simulink model "svpwm"  (R2018a)
settings: Solver=VariableStepDiscrete  StartTime=0.0  StopTime=3  RelTol=1e-3
undefined symbols (not defined in the file): DiscIntNeverNeededParam
libraries: powerlib x16, simulink x3, powerlib_meascontrol x2
settings Model: Creator=HP  LastModifiedBy=HP
settings SolverCC: ZeroCrossAlgorithm=Adaptive
settings DebuggingCC: MaxConsecutiveZCsMsg=none

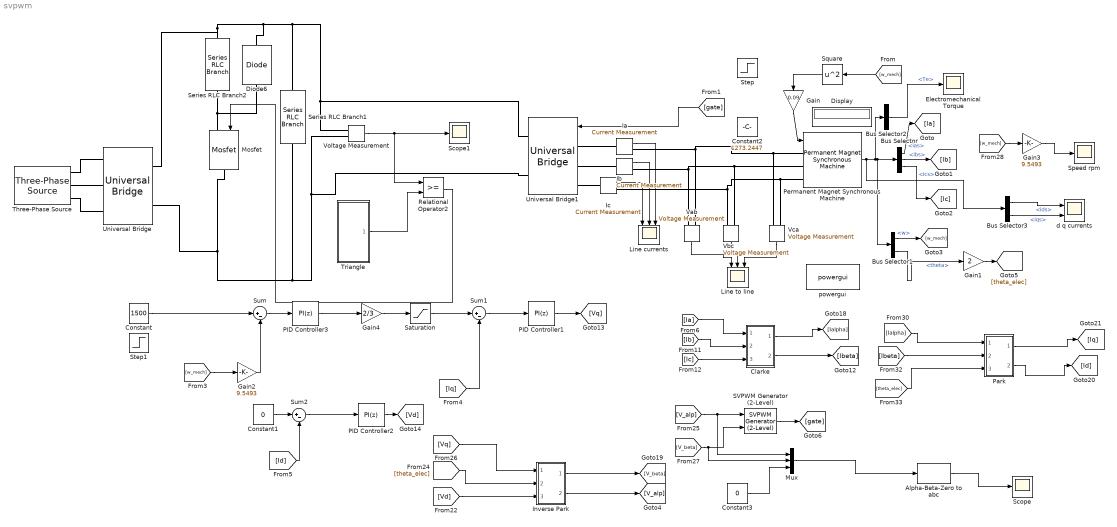
== system svpwm ==
  Alpha-Beta-Zero to abc : powerlib_meascontrol/Transformations/Alpha-Beta-Zero to abc
      settings: SourceProductName=Simscape Power Systems  SourceProductBaseCode=PS
  Bus Selector : BusSelector  OutputSignals=ias,ibs,ics
  Bus Selector1 : BusSelector  OutputSignals=w,theta
  Bus Selector2 : BusSelector  OutputSignals=Te
  Bus Selector3 : BusSelector  OutputSignals=ids,iqs
  Clarke : Subsystem
  Constant : Constant  Value=1500
  Constant1 : Constant  Value=0
  Constant2 : Constant  Value=1273.2447
  Constant3 : Constant  Value=0
  Diode6 : powerlib/Power Electronics/Diode  Ron=0.001  Lon=0  Vf=1  IC=0  UseSnubber=0  Rs=500  Cs=250e-9  Measurements=off
  Display : Display
  Electromechanical Torque : Scope
  Gain : Gain  Gain=0.09
  Gain1 : Gain  Gain=2
  Gain2 : Gain  Gain=9.5493
  Gain3 : Gain  Gain=9.5493
  Gain4 : Gain  Gain=2/3
  Ia : powerlib/Measurements/Current Measurement  PhasorSimulation=off  OutputType=Complex  PSBequivalent=0
  Ib : powerlib/Measurements/Current Measurement  PhasorSimulation=off  OutputType=Complex  PSBequivalent=0
  Ic : powerlib/Measurements/Current Measurement  PhasorSimulation=off  OutputType=Complex  PSBequivalent=0
  Inverse Park : Subsystem
  Line currents : Scope  NumInputPorts=3
  Line to line : Scope  NumInputPorts=3
  Mosfet : powerlib/Power Electronics/Mosfet  Ron=0.1  Lon=0  Rd=0.025  Vfd=0  IC=0  Rs=1e5  Cs=inf  Measurements=off
  Mux : Mux  Inputs=3
  PID Controller1 : simulink/Continuous/PID Controller  Controller=PI  TimeDomain=Discrete-time  SampleTime=-1  IntegratorMethod=Forward Euler  FilterMethod=Forward Euler  Form=Parallel  UseFilter=on  ControllerParametersSource=internal  P=0.1  I=1000  D=0  N=100  InitialConditionSource=internal  InitialConditionForIntegrator=0  InitialConditionForFilter=0  ExternalReset=none  LimitOutput=off  UpperSaturationLimit=inf  LowerSaturationLimit=-inf  LinearizeAsGain=on  AntiWindupMode=none  Kb=1  TrackingMode=off  Kt=1  PParamMin=[]  PParamMax=[]  IParamMin=[]  IParamMax=[]  DParamMin=[]  DParamMax=[]  NParamMin=[]  NParamMax=[]  KbParamMin=[]  KbParamMax=[]  KtParamMin=[]  KtParamMax=[]  POutMin=[]  POutMax=[]  IOutMin=[]  IOutMax=[]  DOutMin=[]  DOutMax=[]  NOutMin=[]  NOutMax=[]  KbOutMin=[]  KbOutMax=[]  KtOutMin=[]  KtOutMax=[]  IntegratorOutMin=[]  IntegratorOutMax=[]  FilterOutMin=[]  FilterOutMax=[]  SumOutMin=[]  SumOutMax=[]  SumI1OutMin=[]  SumI1OutMax=[]  SumI2OutMin=[]  SumI2OutMax=[]  SumI3OutMin=[]  SumI3OutMax=[]  SumDOutMin=[]  SumDOutMax=[]  SaturationOutMin=[]  SaturationOutMax=[]  IntegratorContinuousStateAttributes=''  IntegratorStateMustResolveToSignalObject=off  IntegratorRTWStateStorageClass=Auto  FilterContinuousStateAttributes=''  FilterStateMustResolveToSignalObject=off  FilterRTWStateStorageClass=Auto  DifferentiatorICPrevScaledInput=0  DifferentiatorOutMin=[]  DifferentiatorOutMax=[]  FilterDiffOutCoefMin=[]  FilterDiffOutCoefMax=[]  SumDenOutMin=[]  SumDenOutMax=[]  SumNumOutMin=[]  SumNumOutMax=[]  ReciprocalOutMin=[]  ReciprocalOutMax=[]  DivideOutMin=[]  DivideOutMax=[]  TunerSelectOption=Transfer Function Based (PID Tuner App)
  PID Controller2 : simulink/Continuous/PID Controller  Controller=PI  TimeDomain=Discrete-time  SampleTime=-1  IntegratorMethod=Forward Euler  FilterMethod=Forward Euler  Form=Parallel  UseFilter=on  ControllerParametersSource=internal  P=0.1  I=1000  D=0  N=100  InitialConditionSource=internal  InitialConditionForIntegrator=0  InitialConditionForFilter=0  ExternalReset=none  LimitOutput=off  UpperSaturationLimit=inf  LowerSaturationLimit=-inf  LinearizeAsGain=on  AntiWindupMode=none  Kb=1  TrackingMode=off  Kt=1  PParamMin=[]  PParamMax=[]  IParamMin=[]  IParamMax=[]  DParamMin=[]  DParamMax=[]  NParamMin=[]  NParamMax=[]  KbParamMin=[]  KbParamMax=[]  KtParamMin=[]  KtParamMax=[]  POutMin=[]  POutMax=[]  IOutMin=[]  IOutMax=[]  DOutMin=[]  DOutMax=[]  NOutMin=[]  NOutMax=[]  KbOutMin=[]  KbOutMax=[]  KtOutMin=[]  KtOutMax=[]  IntegratorOutMin=[]  IntegratorOutMax=[]  FilterOutMin=[]  FilterOutMax=[]  SumOutMin=[]  SumOutMax=[]  SumI1OutMin=[]  SumI1OutMax=[]  SumI2OutMin=[]  SumI2OutMax=[]  SumI3OutMin=[]  SumI3OutMax=[]  SumDOutMin=[]  SumDOutMax=[]  SaturationOutMin=[]  SaturationOutMax=[]  IntegratorContinuousStateAttributes=''  IntegratorStateMustResolveToSignalObject=off  IntegratorRTWStateStorageClass=Auto  FilterContinuousStateAttributes=''  FilterStateMustResolveToSignalObject=off  FilterRTWStateStorageClass=Auto  DifferentiatorICPrevScaledInput=0  DifferentiatorOutMin=[]  DifferentiatorOutMax=[]  FilterDiffOutCoefMin=[]  FilterDiffOutCoefMax=[]  SumDenOutMin=[]  SumDenOutMax=[]  SumNumOutMin=[]  SumNumOutMax=[]  ReciprocalOutMin=[]  ReciprocalOutMax=[]  DivideOutMin=[]  DivideOutMax=[]  TunerSelectOption=Transfer Function Based (PID Tuner App)
  PID Controller3 : simulink/Continuous/PID Controller  Controller=PI  TimeDomain=Discrete-time  SampleTime=-1  IntegratorMethod=Forward Euler  FilterMethod=Forward Euler  Form=Parallel  UseFilter=on  ControllerParametersSource=internal  P=1000  I=1  D=0  N=100  InitialConditionSource=internal  InitialConditionForIntegrator=0  InitialConditionForFilter=0  ExternalReset=none  LimitOutput=off  UpperSaturationLimit=inf  LowerSaturationLimit=-inf  LinearizeAsGain=on  AntiWindupMode=none  Kb=1  TrackingMode=off  Kt=1  PParamMin=[]  PParamMax=[]  IParamMin=[]  IParamMax=[]  DParamMin=[]  DParamMax=[]  NParamMin=[]  NParamMax=[]  KbParamMin=[]  KbParamMax=[]  KtParamMin=[]  KtParamMax=[]  POutMin=[]  POutMax=[]  IOutMin=[]  IOutMax=[]  DOutMin=[]  DOutMax=[]  NOutMin=[]  NOutMax=[]  KbOutMin=[]  KbOutMax=[]  KtOutMin=[]  KtOutMax=[]  IntegratorOutMin=[]  IntegratorOutMax=[]  FilterOutMin=[]  FilterOutMax=[]  SumOutMin=[]  SumOutMax=[]  SumI1OutMin=[]  SumI1OutMax=[]  SumI2OutMin=[]  SumI2OutMax=[]  SumI3OutMin=[]  SumI3OutMax=[]  SumDOutMin=[]  SumDOutMax=[]  SaturationOutMin=[]  SaturationOutMax=[]  IntegratorContinuousStateAttributes=''  IntegratorStateMustResolveToSignalObject=off  IntegratorRTWStateStorageClass=Auto  FilterContinuousStateAttributes=''  FilterStateMustResolveToSignalObject=off  FilterRTWStateStorageClass=Auto  DifferentiatorICPrevScaledInput=0  DifferentiatorOutMin=[]  DifferentiatorOutMax=[]  FilterDiffOutCoefMin=[]  FilterDiffOutCoefMax=[]  SumDenOutMin=[]  SumDenOutMax=[]  SumNumOutMin=[]  SumNumOutMax=[]  ReciprocalOutMin=[]  ReciprocalOutMax=[]  DivideOutMin=[]  DivideOutMax=[]  TunerSelectOption=Transfer Function Based (PID Tuner App)
  Park : Subsystem
  Permanent Magnet Synchronous Machine : powerlib/Machines/Permanent Magnet Synchronous Machine  NbPhases=3  FluxDistribution=Sinusoidal  RotorType=Round  MechanicalLoad=Torque Tm  PresetModel=No  ShowDetailedParameters=on  MeasurementBus=on  Resistance=0.016  Inductance=8.5e-3  dqInductances=[8.5e-3,8.5e-3]  La=0.000350  MachineConstant=Flux linkage established by magnets (V.s)  Flux=0.5  VoltageCst=181.3799  TorqueCst=1.5  Flat=120  Mechanical=[250 0 2 0]  PolePairs=4  InitialConditions=[50*pi,0, 0,0]  InitialConditions5ph=[0 0 0 0 0 0]  TsPowergui=0  TsBlock=-1  RefAngle=Aligned with phase A axis (original Park)
      settings: SourceProductName=Simscape Power Systems
  Relational Operator2 : RelationalOperator  OutDataTypeStr=boolean  RndMeth=Simplest
  SVPWM Generator (2-Level) : powerlib_meascontrol/Pulse & Signal Generators/SVPWM Generator (2-Level)  InputType=alpha-beta components  SwitchingPattern=Pattern #1  Fc=5000  ParUref=[0.8 -30 50]  Ts=0
      settings: SourceProductName=Simscape Power Systems  SourceProductBaseCode=PS
  Saturation : Saturate  UpperLimit=1700  LowerLimit=-1700
  Scope : Scope
  Scope1 : Scope
  Series RLC Branch1 : powerlib/Elements/Series RLC Branch  LConnTagsString=__new0  RConnTagsString=__new0  BranchType=C  Resistance=1  Inductance=1e-3  SetiL0=off  InitialCurrent=0  Capacitance=1e-3  Setx0=off  InitialVoltage=0  Measurements=None
  Series RLC Branch2 : powerlib/Elements/Series RLC Branch  LConnTagsString=__new0  RConnTagsString=__new0  BranchType=R  Resistance=0.18  Inductance=1e-3  SetiL0=off  InitialCurrent=0  Capacitance=1e-6  Setx0=off  InitialVoltage=0  Measurements=None
  Speed rpm : Scope
  Square : Math  Operator=square  SaturateOnIntegerOverflow=on
  Step : Step  Time=0.5  Before=2214  After=0  SampleTime=0
  Step1 : Step  Time=0.5  Before=1500  After=-1500  SampleTime=0
  Sum : Sum  Inputs=|+-
  Sum1 : Sum  Inputs=|+-
  Sum2 : Sum  Inputs=|+-
  Three-Phase Source : powerlib/Electrical Sources/Three-Phase Source  InternalConnection=Yg  VoltagePhases=off  Voltage=400  PhaseAngle=0  Voltage_phases=[25e3 25e3 25e3]/sqrt(3)  PhaseAngles_phases=[0 -120 +120]  Frequency=50  NonIdealSource=off  SpecifyImpedance=off  Resistance=0.8929  Inductance=16.58e-3  ShortCircuitLevel=100e6  BaseVoltage=25e3  XRratio=7  BusType=swing  Pref=10e3  Qref=0  Prefabc=[10e3, 10e3, 10e3]  Qrefabc=[0, 0, 0]  Qmin=-inf  Qmax=inf
  Triangle : Subsystem
  Universal Bridge : powerlib/Power Electronics/Universal Bridge  Arms=3  SnubberResistance=1e5  SnubberCapacitance=inf  Device=Diodes  Ron=1e-3  Lon=0  ForwardVoltages="[  0  0  ]"  ForwardVoltage=0  GTOparameters=[ 10e-6 , 20e-6 ]  IGBTparameters=[ 1e-6 , 2e-6 ]  Measurements=None  Measurements_2=None  converterType=Rectifier
  Universal Bridge1 : powerlib/Power Electronics/Universal Bridge  Arms=3  SnubberResistance=1e5  SnubberCapacitance=inf  Device=IGBT / Diodes  Ron=1e-3  Lon=0  ForwardVoltages="[  0  0  ]"  ForwardVoltage=0  GTOparameters=[ 10e-6 , 20e-6 ]  IGBTparameters=[ 1e-6 , 2e-6 ]  Measurements=None  Measurements_2=None  converterType=Rectifier
  Vab : powerlib/Measurements/Voltage Measurement  PhasorSimulation=off  OutputType=Complex  PSBequivalent=0
  Vbc : powerlib/Measurements/Voltage Measurement  PhasorSimulation=off  OutputType=Complex  PSBequivalent=0
  Vca : powerlib/Measurements/Voltage Measurement  PhasorSimulation=off  OutputType=Complex  PSBequivalent=0
  Voltage Measurement : powerlib/Measurements/Voltage Measurement  PhasorSimulation=off  OutputType=Complex  PSBequivalent=0
  d q currents : Scope  NumInputPorts=2
  powergui : powerlib/powergui  Priority=1  SimulationMode=Discrete  SampleTime=1e-5  frequency=60  Iterations=50  frequencyindice=0  Pbase=100e6  ErrMax=1e-4  UnitsV=kV  UnitsW=MW  buscounter=0  FunctionMessages=off  echomessages=off  EnableUseOfTLC=off  CurrentSourceSwitches=off  DisableSnubberDevices=off  DisableRonSwitches=off  DisableVfSwitches=off  DisplayEquations=off  SolverType=Tustin/Backward Euler (TBE)  Interpol=off  ExternalGateDelay=off  methode=off  Ts=100  x0status=blocks  SPID=on  SwTol=0  HookPort=off  RestoreLinks=warning  ResistiveCurrentMeasurement=off  Frange=[0:2:500]  Ylog=off  Xlog=on  ShowGrid=off  save=off  variable=ZData  structure=line_currents  ZoomFFT=off  StartTime=1.7  cycles=10  DisplayStyle=1  fundamental=50  FreqAxis=on  MaxFrequency=500  frequencyindicesteady=1  RmsSteady=1  display=off
  wires:
  [w_mech] -> Square/1
  Square/1 -> Gain/1
  Permanent Magnet Synchronous Machine/1 -> Bus Selector3/1, Bus Selector2/1, Bus Selector1/1, Bus Selector/1
  Bus Selector/1 -> [Ia]  "<ias>"
  Bus Selector/2 -> [Ib]  "<ibs>"
  Bus Selector/3 -> [Ic]  "<ics>"
  Bus Selector2/1 -> Electromechanical Torque/1  "<Te>"
  Bus Selector1/1 -> [w_mech]  "<w>"
  Bus Selector1/2 -> Gain1/1  "<theta>"
  Gain1/1 -> [theta_elec]
  SVPWM Generator (2-Level)/1 -> [gate]
  [w_mech] -> Gain2/1
  Gain2/1 -> Sum/2
  Sum/1 -> PID Controller3/1
  PID Controller3/1 -> Gain4/1
  Gain4/1 -> Saturation/1
  Saturation/1 -> Sum1/1
  Sum1/1 -> PID Controller1/1
  Constant1/1 -> Sum2/1
  [Id] -> Sum2/2
  PID Controller1/1 -> [Vq]
  PID Controller2/1 -> [Vd]
  [V_alp] -> Mux/1, SVPWM Generator (2-Level)/1
  [V_beta] -> Mux/2, SVPWM Generator (2-Level)/2
  [w_mech] -> Gain3/1
  Gain3/1 -> Speed rpm/1
  [Ia] -> Clarke/1(In1)
  [Ib] -> Clarke/2(In2)
  [Ic] -> Clarke/3(In3)
  Clarke/1(Ialpha) -> [Ialpha]
  Clarke/2(Ibeta) -> [Ibeta]
  [Ialpha] -> Park/1(In1)
  [Ibeta] -> Park/2(In2)
  [theta_elec] -> Park/3(In3)
  [Vq] -> Inverse Park/1(In1)
  [theta_elec] -> Inverse Park/2(In2)
  [Vd] -> Inverse Park/3(In3)
  Inverse Park/1(Out1) -> [V_beta]
  Inverse Park/2(Out2) -> [V_alp]
  Relational Operator2/1 -> Mosfet/1
  Voltage Measurement/1 -> Scope1/1, Relational Operator2/1
  Triangle/1(Triangular) -> Relational Operator2/2
  [gate] -> Universal Bridge1/1
  Vab/1 -> Line to line/1
  Vbc/1 -> Line to line/2
  Vca/1 -> Line to line/3
  Bus Selector3/1 -> d q currents/1  "<ids>"
  Bus Selector3/2 -> d q currents/2  "<iqs>"
  Ia/1 -> Line currents/3
  Ib/1 -> Line currents/2
  Ic/1 -> Line currents/1
  Sum2/1 -> PID Controller2/1
  [Iq] -> Sum1/2
  Park/1(Out1) -> [Iq]
  Park/2(Out2) -> [Id]
  Constant/1 -> Sum/1
  Constant3/1 -> Mux/3
  Mux/1 -> Alpha-Beta-Zero to abc/1
  Gain/1 -> Permanent Magnet Synchronous Machine/1
  Alpha-Beta-Zero to abc/1 -> Scope/1
  connections:
  Series RLC Branch1/RConn1 -- Universal Bridge/RConn2 -- Mosfet/RConn1 -- Universal Bridge1/RConn2 -- Voltage Measurement/LConn2
  Voltage Measurement/LConn1 -- Universal Bridge1/RConn1 -- Series RLC Branch1/LConn1 -- Universal Bridge/RConn1 -- Series RLC Branch2/LConn1 -- Diode6/RConn1
  Three-Phase Source/RConn1 -- Universal Bridge/LConn1
  Three-Phase Source/RConn2 -- Universal Bridge/LConn2
  Three-Phase Source/RConn3 -- Universal Bridge/LConn3
  Series RLC Branch2/RConn1 -- Mosfet/LConn1 -- Diode6/LConn1
  Vab/LConn1 -- Ia/RConn1 -- Vca/LConn2 -- Permanent Magnet Synchronous Machine/LConn1
  Vab/LConn2 -- Ib/RConn1 -- Permanent Magnet Synchronous Machine/LConn2 -- Vbc/LConn1
  Permanent Magnet Synchronous Machine/LConn3 -- Ic/RConn1 -- Vbc/LConn2 -- Vca/LConn1
  Ia/LConn1 -- Universal Bridge1/LConn1
  Universal Bridge1/LConn2 -- Ib/LConn1
  Ic/LConn1 -- Universal Bridge1/LConn3

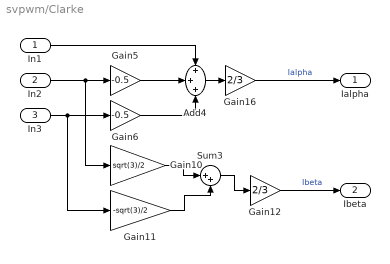
== system svpwm/Clarke ==
  In1 : Inport
  In2 : Inport  Port=2
  In3 : Inport  Port=3
  Add4 : Sum  Inputs=+++
  Gain10 : Gain  Gain=sqrt(3)/2
  Gain11 : Gain  Gain=-sqrt(3)/2
  Gain12 : Gain  Gain=2/3
  Gain16 : Gain  Gain=2/3
  Gain5 : Gain  Gain=-0.5
  Gain6 : Gain  Gain=-0.5
  Sum3 : Sum  Inputs=|++
  Ialpha : Outport
  Ibeta : Outport  Port=2
  wires:
  In2/1 -> Gain10/1, Gain5/1
  Add4/1 -> Gain16/1
  Gain10/1 -> Sum3/1
  Gain6/1 -> Add4/3
  In3/1 -> Gain11/1, Gain6/1
  Sum3/1 -> Gain12/1
  Gain5/1 -> Add4/2
  In1/1 -> Add4/1
  Gain11/1 -> Sum3/2
  Gain12/1 -> Ibeta/1  "Ibeta"
  Gain16/1 -> Ialpha/1  "Ialpha"

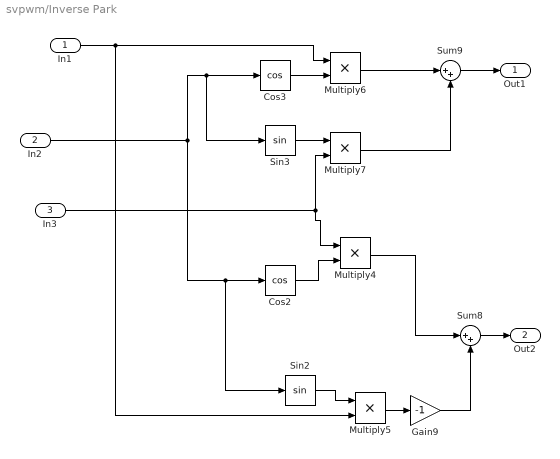
== system svpwm/Inverse Park ==
  In1 : Inport
  In2 : Inport  Port=2
  In3 : Inport  Port=3
  Cos2 : Trigonometry  Operator=cos
  Cos3 : Trigonometry  Operator=cos
  Gain9 : Gain  Gain=-1
  Multiply{4..7} (4 alike) : Product
  Sin2 : Trigonometry
  Sin3 : Trigonometry
  Sum8 : Sum  Inputs=|++
  Sum9 : Sum  Inputs=|++
  Out1 : Outport
  Out2 : Outport  Port=2
  wires:
  Cos2/1 -> Multiply4/2
  In1/1 -> Multiply5/2, Multiply6/1
  Sum9/1 -> Out1/1
  Sin2/1 -> Multiply5/1
  In2/1 -> Sin3/1, Cos3/1, Sin2/1, Cos2/1
  In3/1 -> Multiply4/1, Multiply7/2
  Cos3/1 -> Multiply6/2
  Sin3/1 -> Multiply7/1
  Multiply5/1 -> Gain9/1
  Multiply4/1 -> Sum8/1
  Gain9/1 -> Sum8/2
  Multiply7/1 -> Sum9/2
  Multiply6/1 -> Sum9/1
  Sum8/1 -> Out2/1

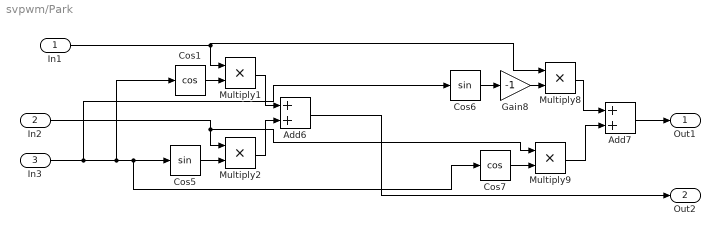
== system svpwm/Park ==
  In1 : Inport
  In2 : Inport  Port=2
  In3 : Inport  Port=3
  Add6 : Sum
  Add7 : Sum
  Cos1 : Trigonometry  Operator=cos
  Cos5 : Trigonometry
  Cos6 : Trigonometry
  Cos7 : Trigonometry  Operator=cos
  Gain8 : Gain  Gain=-1
  Multiply{1..2,8..9} (4 alike) : Product
  Out1 : Outport
  Out2 : Outport  Port=2
  wires:
  Cos7/1 -> Multiply9/2
  In3/1 -> Cos6/1, Cos1/1, Cos7/1, Cos5/1
  In1/1 -> Multiply8/1, Multiply1/1
  Cos1/1 -> Multiply1/2
  Cos6/1 -> Gain8/1
  Add6/1 -> Out2/1
  In2/1 -> Multiply9/1, Multiply2/1
  Gain8/1 -> Multiply8/2
  Multiply9/1 -> Add7/2
  Cos5/1 -> Multiply2/2
  Multiply8/1 -> Add7/1
  Multiply2/1 -> Add6/2
  Multiply1/1 -> Add6/1
  Add7/1 -> Out1/1

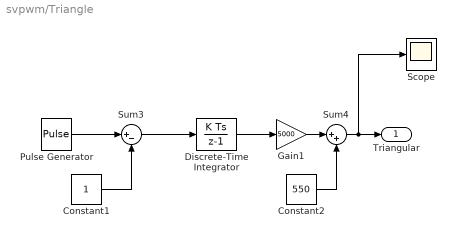
== system svpwm/Triangle ==
  Constant1 : Constant
  Constant2 : Constant  Value=550
  Discrete-Time Integrator : DiscreteIntegrator  SampleTime=-1  ICPrevOutput=DiscIntNeverNeededParam  ICPrevScaledInput=DiscIntNeverNeededParam
  Gain1 : Gain  Gain=5000
  Pulse Generator : DiscretePulseGenerator  PulseType=Time based  Amplitude=2  Period=1/5000  PulseWidth=50
  Scope : Scope
  Sum3 : Sum  Inputs=|+-
  Sum4 : Sum  Inputs=|++
  Triangular : Outport
  wires:
  Constant1/1 -> Sum3/2
  Gain1/1 -> Sum4/1
  Constant2/1 -> Sum4/2
  Sum4/1 -> Scope/1, Triangular/1
  Sum3/1 -> Discrete-Time Integrator/1
  Pulse Generator/1 -> Sum3/1
  Discrete-Time Integrator/1 -> Gain1/1
